simulink model "Train"  (R2024a)
settings: Solver=FixedStepDiscrete  StartTime=0.0  StopTime=400  FixedStep=Ts  RelTol=1e-3
values from neighbouring files (symbols this model uses):
  a = exp(-plant.Ts/plant.tau)    [Main.m]
  b = plant.K*(1 - a)    [Main.m]
  g = b * 1.7    [Main.m]
  XKP0 = 0    [Main.m]
  Y0 = 0  +  5*rand()    [Main.m]
undefined symbols (not defined in the file or in its folder): beta1, beta2, Dmax, Emax, eta, fD, fS, L, q, rho, Ts, UMAX, Umax, Ymax
libraries: simulink x2, rllib x1
settings Model: Creator=admin  LastModifiedBy=admin

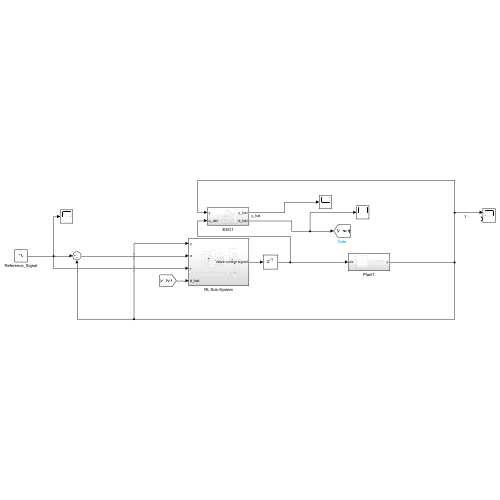
[thumbnail: Simulink's stored preview of the top-level diagram]
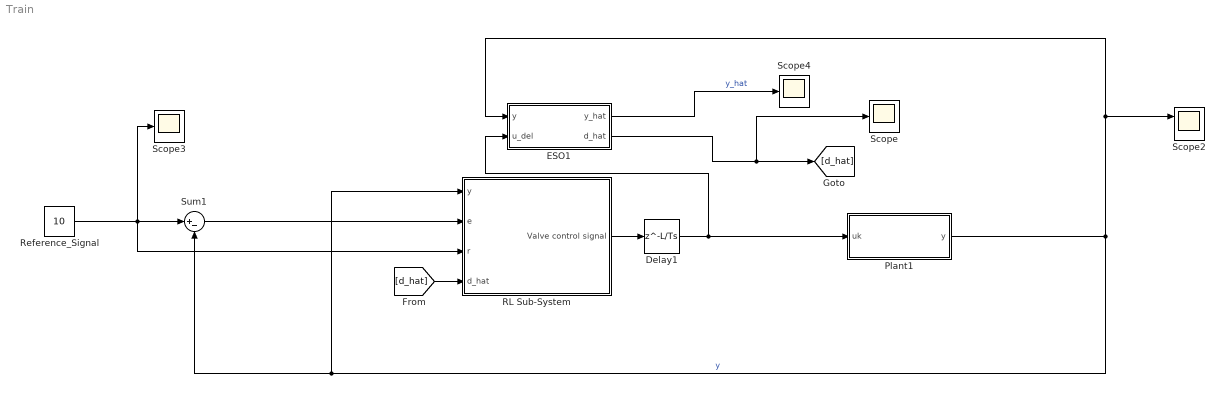
== system Train ==
  Delay1 : Delay  DelayLength=L/Ts
  ESO1 : Subsystem
  Plant1 : Subsystem
  RL Sub-System : Subsystem
  Reference_Signal : Constant  Value=10
  Scope : Scope
  Scope2 : Scope  NumInputPorts=2
  Scope3 : Scope
  Scope4 : Scope
  Sum1 : Sum  Inputs=|+-
  wires:
  Delay1/1 -> ESO1/2(u_del), Plant1/1(uk)
  Reference_Signal/1 -> RL Sub-System/3(r), Sum1/1, Scope3/1
  Plant1/1(y) -> ESO1/1(y), Scope2/1, RL Sub-System/1(y), Sum1/2  "y"
  RL Sub-System/1(Valve control signal) -> Delay1/1
  Sum1/1 -> RL Sub-System/2(e)
  ESO1/2(d_hat) -> Scope/1, [d_hat]
  [d_hat] -> RL Sub-System/4(d_hat)
  ESO1/1(y_hat) -> Scope4/1  "y_hat"

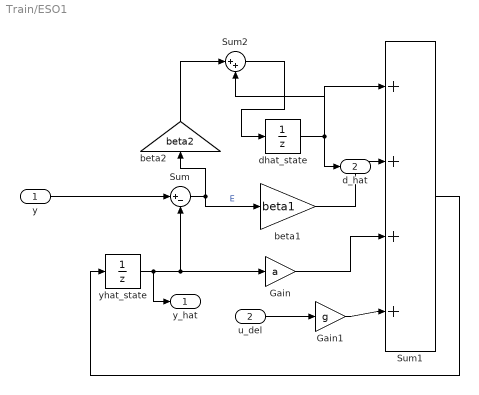
== system Train/ESO1 ==
  y : Inport
  u_del : Inport  Port=2
  Gain : Gain  Gain=a
  Gain1 : Gain  Gain=g
  Sum : Sum  Inputs=|+-
  Sum1 : Sum  Inputs=|++++
  Sum2 : Sum  Inputs=|++
  beta1 : Gain  Gain=beta1
  beta2 : Gain  Gain=beta2
  dhat_state : UnitDelay  SampleTime=-1  HasFrameUpgradeWarning=on
  yhat_state : UnitDelay  SampleTime=-1  HasFrameUpgradeWarning=on
  y_hat : Outport
  d_hat : Outport  Port=2
  wires:
  yhat_state/1 -> y_hat/1, Gain/1, Sum/2
  y/1 -> Sum/1
  Sum/1 -> beta2/1, beta1/1  "E"
  u_del/1 -> Gain1/1
  Sum1/1 -> yhat_state/1
  Gain1/1 -> Sum1/4
  Gain/1 -> Sum1/3
  beta1/1 -> Sum1/2
  dhat_state/1 -> d_hat/1, Sum1/1, Sum2/2
  beta2/1 -> Sum2/1
  Sum2/1 -> dhat_state/1

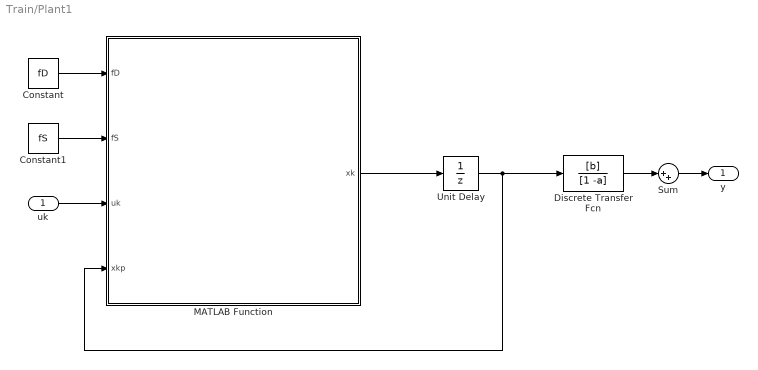
== system Train/Plant1 ==
  uk : Inport
  Constant : Constant  Value=fD
  Constant1 : Constant  Value=fS
  Discrete Transfer Fcn : DiscreteTransferFcn  Numerator=[b]  Denominator=[1 -a]  InitialStates=Y0
  MATLAB Function : MATLAB Function  TreatAsAtomicUnit=on
  Sum : Sum  Inputs=|++
  Unit Delay : UnitDelay  InitialCondition=XKP0  SampleTime=Ts  HasFrameUpgradeWarning=on
  y : Outport
  wires:
  MATLAB Function/1(xk) -> Unit Delay/1
  Unit Delay/1 -> MATLAB Function/4(xkp), Discrete Transfer Fcn/1
  Constant/1 -> MATLAB Function/1(fD)
  Constant1/1 -> MATLAB Function/2(fS)
  uk/1 -> MATLAB Function/3(uk)
  Discrete Transfer Fcn/1 -> Sum/1
  Sum/1 -> y/1

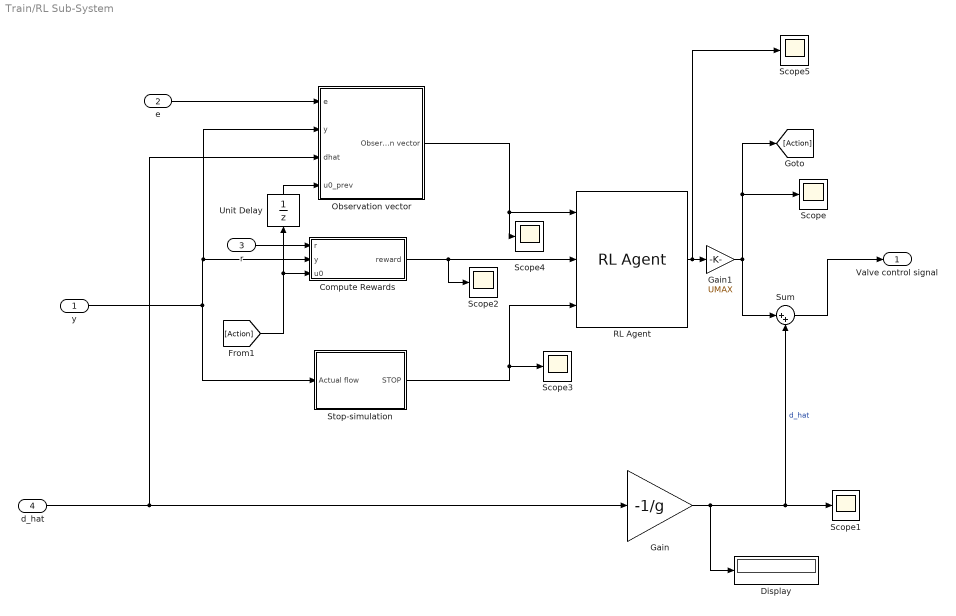
== system Train/RL Sub-System ==
  y : Inport
  e : Inport  Port=2
  r : Inport  Port=3
  d_hat : Inport  Port=4
  Compute Rewards : Subsystem
  Display : Display
  Gain : Gain  Gain=-1/g
  Gain1 : Gain  Gain=UMAX
  Observation vector : Subsystem
  RL Agent : rllib/RL Agent  Agent=agent  ExternalActionAsInput=off  ProvideLastAction=off  ProvideCumRwd=off  TreatAsDirectFeedthrough=on  UseStrictObservationDataTypes=off
  Scope{,1..5} (6 alike) : Scope
  Stop-simulation : Subsystem
  Sum : Sum  Inputs=|++
  Unit Delay : UnitDelay  SampleTime=-1  HasFrameUpgradeWarning=on
  Valve control signal : Outport  VectorParamsAs1DForOutWhenUnconnected=off
  wires:
  Unit Delay/1 -> Observation vector/4(u0_prev)
  r/1 -> Compute Rewards/1(r)
  Compute Rewards/1(reward) -> Scope2/1, RL Agent/2
  e/1 -> Observation vector/1(e)
  Observation vector/1(Observation vector) -> Scope4/1, RL Agent/1
  Stop-simulation/1(STOP) -> Scope3/1, RL Agent/3
  [Action] -> Unit Delay/1, Compute Rewards/3(u0)
  y/1 -> Observation vector/2("y "), Compute Rewards/2(y), Stop-simulation/1(Actual flow)
  d_hat/1 -> Observation vector/3(dhat), Gain/1
  Gain/1 -> Display/1, Scope1/1, Sum/2  "d_hat"
  Sum/1 -> Valve control signal/1
  RL Agent/1 -> Scope5/1, Gain1/1
  Gain1/1 -> [Action], Scope/1, Sum/1

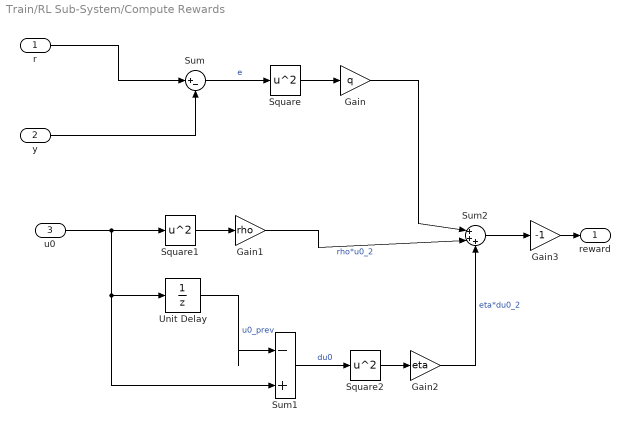
== system Train/RL Sub-System/Compute Rewards ==
  r : Inport
  y : Inport  Port=2
  u0 : Inport  Port=3
  Gain : Gain  Gain=q
  Gain1 : Gain  Gain=rho
  Gain2 : Gain  Gain=eta
  Gain3 : Gain  Gain=-1
  Square : Math  Operator=square
  Square1 : Math  Operator=square
  Square2 : Math  Operator=square
  Sum : Sum  Inputs=|+-
  Sum1 : Sum  Inputs=|-+
  Sum2 : Sum  Inputs=|+++
  Unit Delay : UnitDelay  SampleTime=-1  HasFrameUpgradeWarning=on
  reward : Outport
  wires:
  Sum2/1 -> Gain3/1
  Unit Delay/1 -> Sum1/1  "u0_prev"
  Gain2/1 -> Sum2/3  "eta*du0_2"
  Gain/1 -> Sum2/1
  r/1 -> Sum/1
  Sum1/1 -> Square2/1  "du0"
  u0/1 -> Sum1/2, Unit Delay/1, Square1/1
  Gain3/1 -> reward/1
  y/1 -> Sum/2
  Square2/1 -> Gain2/1
  Gain1/1 -> Sum2/2  "rho*u0_2"
  Square/1 -> Gain/1
  Sum/1 -> Square/1  "e"
  Square1/1 -> Gain1/1

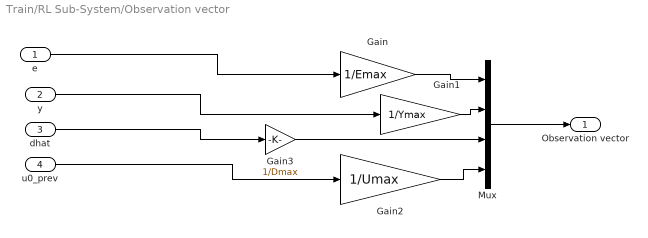
== system Train/RL Sub-System/Observation vector ==
  e : Inport
  "y " : Inport  Port=2
  dhat : Inport  Port=3
  u0_prev : Inport  Port=4
  Gain : Gain  Gain=1/Emax
  Gain1 : Gain  Gain=1/Ymax
  Gain2 : Gain  Gain=1/Umax
  Gain3 : Gain  Gain=1/Dmax
  Mux : Mux
  Observation vector : Outport
  wires:
  Mux/1 -> Observation vector/1
  e/1 -> Gain/1
  "y "/1 -> Gain1/1
  u0_prev/1 -> Gain2/1
  Gain/1 -> Mux/1
  Gain1/1 -> Mux/2
  dhat/1 -> Gain3/1
  Gain2/1 -> Mux/4
  Gain3/1 -> Mux/3

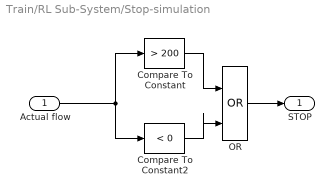
== system Train/RL Sub-System/Stop-simulation ==
  Actual flow : Inport
  Compare To Constant : simulink/Logic and Bit Operations/Compare To Constant  relop=>  const=200  OutDataTypeStr=boolean
  Compare To Constant2 : simulink/Logic and Bit Operations/Compare To Constant  relop=<  const=0  OutDataTypeStr=boolean
  OR : Logic  Operator=OR  IconShape=distinctive  AllPortsSameDT=off  OutDataTypeStr=boolean
  STOP : Outport  VectorParamsAs1DForOutWhenUnconnected=off
  wires:
  Compare To Constant/1 -> OR/1
  Actual flow/1 -> Compare To Constant/1, Compare To Constant2/1
  Compare To Constant2/1 -> OR/2
  OR/1 -> STOP/1

== matlab function Train/Plant1/MATLAB Function ==
  data: fD input; xk output; fS input; uk input; xkp input
function xk = FrictionMap(fD, fS, uk, xkp)
%#codegen
t_xk = 0.0;
v = 1.7*uk - xkp;
if v >  fS
    t_xk = 1.7*uk - fD;
elseif v < -fS
    t_xk = 1.7*uk + fD;
else
    t_xk = xkp;
end
xk = t_xk;
end
